simulink model "Joystick"  (Simulink 7.7)
settings: Solver=ode4  StartTime=0.0  StopTime=inf  FixedStep=sample_time  RelTol=1e-3
InitFcn:
  | sample_time=0.01;
libraries: vrlib x2, utility x1
settings Model: Creator=ttcl3  LastModifiedBy=CHIEW
settings SolverCC: MaxConsecutiveMinStep=auto
settings DebuggingCC: MultiTaskRateTransMsg=warning

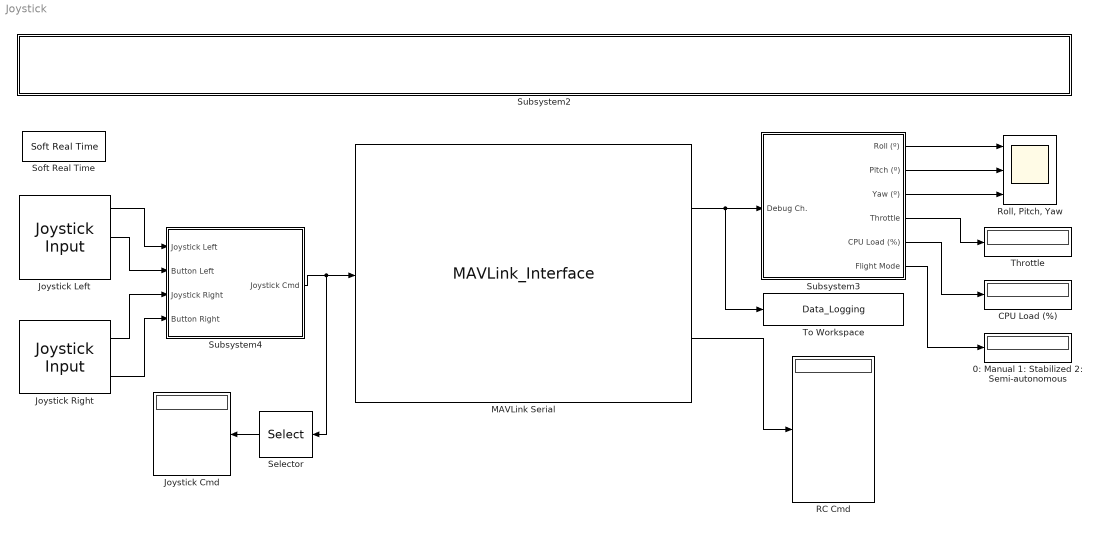
== system Joystick ==
  0: Manual 1: Stabilized 2: Semi-autonomous : Display
  CPU Load (%) : Display
  Joystick Cmd : Display
  Joystick Left : vrlib/Joystick Input  joyid=2  adjustports=on  forcefeed=off
  Joystick Right : vrlib/Joystick Input  joyid=1  adjustports=on  forcefeed=off
  MAVLink Serial : S-Function  FunctionName=MAVLink_Interface  Parameters=COM_Port,Baud_Rate,MSG_INPUT,MSG_OUTPUT  EnableBusSupport=off  mask{COM_Port='COM8', Baud_Rate=57600, HEART_BEAT=off, ATTITUDE_OUT=on, RAW_IMU=off, POSITION_OUT=off, VFR_HUD=off, RC_SCALED=on, SERVO_OUT_RAW=off, VICON_XYZ_RPY_Output=off, SET_MODE=off, DATA_STREAM=off, ATTITUDE_COMMAND=off, ATTITUDE_IN=off, GPS_RAW_IN=off, VFR_HUD_IN=off, VICON_XYZ_RPY=on, VICON_VEL=off, POSITION_DESIRED=off}
      mask prompts: COM_Port "COM Port"; Baud_Rate "Baud Rate"; HEART_BEAT "HEART BEAT"; ATTITUDE_OUT "ATTITUDE"; RAW_IMU "RAW IMU"; POSITION_OUT "GLOBAL POSITION"; VFR_HUD "VFR HUD"; RC_SCALED "RC CHANNELS SCALED"; SERVO_OUT_RAW "SERVO OUTPUT RAW"; VICON_XYZ_RPY_Output "VICON Output"; SET_MODE "SET MODE"; DATA_STREAM "REQUEST DATA STREAM"; ATTITUDE_COMMAND "ATTITUDE COMMAND"; ATTITUDE_IN "ATTITUDE (HIL)"; GPS_RAW_IN "GPS RAW (HIL)"; VFR_HUD_IN "AIRSPEED (HIL)"; VICON_XYZ_RPY "VICON POSITION"; VICON_VEL "VICON SPEED"; POSITION_DESIRED "Position Desired"
      mask init:
      | MSG_ID_NUM_INPUT = [uint8(11) uint8(66) uint8(59) uint8(30) uint8(32) uint8(73) uint8(104) uint8(103) uint8(50)];
      | MSG_ID_NAME_INPUT = [SET_MODE DATA_STREAM ATTITUDE_COMMAND ATTITUDE_IN GPS_RAW_IN VFR_HUD_IN VICON_XYZ_RPY VICON_VEL POSITION_DESIRED];
      | 
      | MSG_ID_NUM_OUTPUT = [uint8(0) uint8(30) uint8(27) uint8(73) uint8(74) uint8(34) uint8(37) uint8(104)];
      | MSG_ID_NAME_OUTPUT = [HEART_BEAT ATTITUDE_OUT RAW_IMU VFR_HUD POSITION_OUT RC_SCALED SERVO_OUT_RAW VICON_XYZ_RPY_Output];
      | 
      | idx_input = find(MSG_ID_NAME_INPUT);
      | MSG_INPUT = MSG_ID_NUM_INPUT(idx_input);
      | 
      | idx_output = find(MSG_ID_NAME_OUTPUT);
      | MSG_OUTPUT = MSG_ID_NUM_OUTPUT(idx_output);
      mask TabNameString: Setting,Setting,Output Message,Output Message,Output Message,Output Message,Output Message,Output Message,Output Message,Output Message,Input Message,Input Message,Input Message,Input Message,Input Message,Input Message,Input Message,Input Message,Input Message
      mask Display:
      | % Block image
      | image(imread('10-inch Quad Heat Map.png'));
      | 
      | %Label block
      | fprintf('MAVLink Serial\n%s\n%dbps', COM_Port,  Baud_Rate)
      | 
      | 
      | %Label input ports
      | 
      | in = 1;
      | if (SET_MODE == 1)
      |     port_label('input', in, 'SET MODE');
      |     in = in + 1;
      | end
      | if (DATA_STREAM == 1)
      |     port_label('input', in, 'REQUEST DATA STREAM');
      |     in = in + 1;
      | end
      | if (ATTITUDE_COMMAND == 1)
      |     port_label('input', in, 'ATTITUDE COMMAND');
      |     in = in + 1;
      | end
      | if (ATTITUDE_IN == 1)
      |     port_label('input', in, 'ATTITUDE (HIL)');
      |     in = in + 1;
      | end
      | if (GPS_RAW_IN == 1)
      |     port_label('input', in, 'GPS RAW (HIL)');
      |     in = in + 1;
      | end
      | if (VFR_HUD_IN == 1)
      |     port_label('input', in, 'AIRSPEED (HIL)');
      |     in = in + 1;
      | end
      | if (VICON_XYZ_RPY == 1)
      |     port_label('input', in, 'JOYSTICK CMD');
      |     in = in + 1;
      | end
      | if (VICON_VEL == 1)
      |     port_label('input', in, 'VICON_VEL');
      |     in = in + 1;
      | end
      | 
      | if (POSITION_DESIRED == 1)
      |     port_label('input', in, 'POSITION_DESIRED');
      |     in = in + 1;
      | end
      | 
      | %Label output ports
      | 
      | out = 1;
      | if (HEART_BEAT == 1)
      |     port_label('output', out, 'HEART BEAT');
      |     out = out + 1;
      | end
      | if (ATTITUDE_OUT == 1)
      |     port_label('output', out, 'DEBUG');
      |     out = out + 1;
      | end
      | if (RAW_IMU == 1)
      |     port_label('output', out, 'RAW IMU');
      |     out = out + 1;
      | end
      | if (POSITION_OUT == 1)
      |     port_label('output', out, 'GLOBAL POSITION');
      |     out = out + 1;
      | end
      | if (VFR_HUD == 1)
      |     port_label('output', out, 'VFR HUD');
      |     out = out + 1;
      | end
      | if (RC_SCALED == 1)
      |     port_label('output', out, 'RC CMD');
      |     out = out + 1;
      | end
      | if (SERVO_OUT_RAW == 1)
      |     port_label('output', out, 'SERVO OUTPUT RAW');
      |     out = out + 1;
      | end
      | % weihua, vicon output
      | if (VICON_XYZ_RPY_Output == 1)
      |     port_label('output', out, 'VICON_XYZ_RPY');
      |     out = out + 1;
      | end
  RC Cmd : Display
  "Roll, Pitch, Yaw" : Scope  NumInputPorts=3
      settings: TickLabels=on  TimeRange=24  YMin=-20~-10~-40  YMax=90~90~40  SampleInput=on
  Selector : Selector  InputPortWidth=7  IndexOptions=Index vector (dialog)  Indices=[4:7]  OutputSizes=1
  Soft Real Time : utility/Soft Real Time  x=0.8
  Subsystem2 : Subsystem
      mask Display:
      | %Label block
      | fprintf('NANYANG TECHNOLOGICAL UNIVERSITY')
  Subsystem3 : Subsystem
  Subsystem4 : Subsystem
  Throttle : Display
  To Workspace : ToWorkspace  VariableName=Data_Logging  SampleTime=-1  SaveFormat=Structure With Time
  wires:
  Subsystem4/1(Joystick Cmd) -> MAVLink Serial/1, Selector/1
  Joystick Left/1 -> Subsystem4/1(Joystick Left)
  Joystick Right/1 -> Subsystem4/3(Joystick Right)
  MAVLink Serial/2 -> RC Cmd/1
  Subsystem3/1(Roll (º)) -> "Roll, Pitch, Yaw"/1
  Subsystem3/2(Pitch (º)) -> "Roll, Pitch, Yaw"/2
  Subsystem3/3(Yaw (º)) -> "Roll, Pitch, Yaw"/3
  Subsystem3/4(Throttle) -> Throttle/1
  Subsystem3/5(CPU Load (%)) -> CPU Load (%)/1
  Subsystem3/6(Flight Mode) -> 0: Manual 1: Stabilized 2: Semi-autonomous/1
  Selector/1 -> Joystick Cmd/1
  MAVLink Serial/1 -> Subsystem3/1(Debug Ch.), To Workspace/1
  Joystick Right/2 -> Subsystem4/4(Button Right)
  Joystick Left/2 -> Subsystem4/2(Button Left)

== system Joystick/Subsystem2 ==

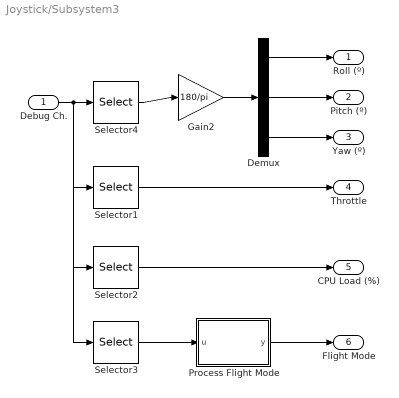
== system Joystick/Subsystem3 ==
  Debug Ch. : Inport
  Demux : Demux  Outputs=3
  Gain2 : Gain  Gain=180/pi
  Process Flight Mode : Stateflow chart  TreatAsAtomicUnit=on
  Selector1 : Selector  InputPortWidth=6  IndexOptions=Index vector (dialog)  Indices=4  OutputSizes=1
  Selector2 : Selector  InputPortWidth=6  IndexOptions=Index vector (dialog)  Indices=5  OutputSizes=1
  Selector3 : Selector  InputPortWidth=6  IndexOptions=Index vector (dialog)  Indices=6  OutputSizes=1
  Selector4 : Selector  InputPortWidth=6  IndexOptions=Index vector (dialog)  Indices=[1 2 3]  OutputSizes=1
  Roll (º) : Outport
  Pitch (º) : Outport  Port=2
  Yaw (º) : Outport  Port=3
  Throttle : Outport  Port=4
  CPU Load (%) : Outport  Port=5
  Flight Mode : Outport  Port=6
  wires:
  Selector4/1 -> Gain2/1
  Gain2/1 -> Demux/1
  Demux/1 -> Roll (º)/1
  Demux/2 -> Pitch (º)/1
  Debug Ch./1 -> Selector4/1, Selector1/1, Selector2/1, Selector3/1
  Demux/3 -> Yaw (º)/1
  Selector1/1 -> Throttle/1
  Selector2/1 -> CPU Load (%)/1
  Selector3/1 -> Process Flight Mode/1(u)
  Process Flight Mode/1(y) -> Flight Mode/1

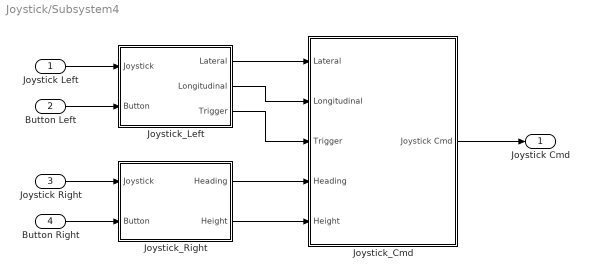
== system Joystick/Subsystem4 ==
  Joystick Left : Inport
  Button Left : Inport  Port=2
  Joystick Right : Inport  Port=3
  Button Right : Inport  Port=4
  Joystick_Cmd : Subsystem
  Joystick_Left : Subsystem
  Joystick_Right : Subsystem
  Joystick Cmd : Outport
  wires:
  Joystick_Right/2(Height) -> Joystick_Cmd/5(Height)
  Joystick_Left/1(Lateral) -> Joystick_Cmd/1(Lateral)
  Joystick Left/1 -> Joystick_Left/1(Joystick)
  Joystick_Cmd/1(Joystick Cmd) -> Joystick Cmd/1
  Joystick Right/1 -> Joystick_Right/1(Joystick)
  Button Right/1 -> Joystick_Right/2(Button)
  Joystick_Left/2(Longitudinal) -> Joystick_Cmd/2(Longitudinal)
  Joystick_Right/1(Heading) -> Joystick_Cmd/4(Heading)
  Button Left/1 -> Joystick_Left/2(Button)
  Joystick_Left/3(Trigger) -> Joystick_Cmd/3(Trigger)

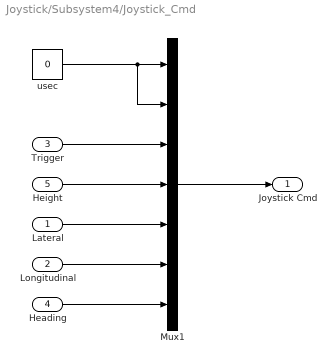
== system Joystick/Subsystem4/Joystick_Cmd ==
  Lateral : Inport
  Longitudinal : Inport  Port=2
  Trigger : Inport  Port=3
  Heading : Inport  Port=4
  Height : Inport  Port=5
  Mux1 : Mux  Inputs=7
  usec : Constant  Value=0  SampleTime=sample_time
  Joystick Cmd : Outport
  wires:
  usec/1 -> Mux1/1, Mux1/2
  Mux1/1 -> Joystick Cmd/1
  Height/1 -> Mux1/4
  Lateral/1 -> Mux1/5
  Longitudinal/1 -> Mux1/6
  Heading/1 -> Mux1/7
  Trigger/1 -> Mux1/3

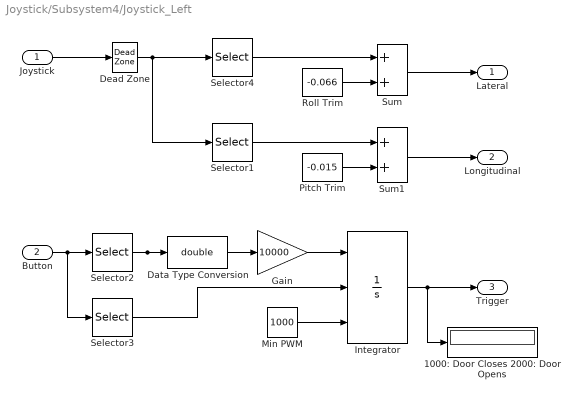
== system Joystick/Subsystem4/Joystick_Left ==
  Joystick : Inport
  Button : Inport  Port=2
  1000: Door Closes 2000: Door Opens : Display
  Data Type Conversion : DataTypeConversion  OutDataTypeStr=double
  Dead Zone : DeadZone  LowerValue=-0.1  UpperValue=0.1  SaturateOnIntegerOverflow=on
  Gain : Gain  Gain=10000
  Integrator : Integrator  ExternalReset=either  InitialConditionSource=external  LimitOutput=on  UpperSaturationLimit=1800  LowerSaturationLimit=1000
  Min PWM : Constant  Value=1000
  Pitch Trim : Constant  Value=-0.015
  Roll Trim : Constant  Value=-0.066
  Selector1 : Selector  InputPortWidth=4  IndexOptions=Index vector (dialog)  Indices=2  OutputSizes=1
  Selector2 : Selector  InputPortWidth=12  IndexOptions=Index vector (dialog)  Indices=1  OutputSizes=1
  Selector3 : Selector  InputPortWidth=12  IndexOptions=Index vector (dialog)  Indices=4  OutputSizes=1
  Selector4 : Selector  InputPortWidth=4  IndexOptions=Index vector (dialog)  Indices=1  OutputSizes=1
  Sum : Sum
  Sum1 : Sum
  Lateral : Outport
  Longitudinal : Outport  Port=2
  Trigger : Outport  Port=3
  wires:
  Joystick/1 -> Dead Zone/1
  Roll Trim/1 -> Sum/2
  Pitch Trim/1 -> Sum1/2
  Dead Zone/1 -> Selector4/1, Selector1/1
  Selector4/1 -> Sum/1
  Selector1/1 -> Sum1/1
  Sum/1 -> Lateral/1
  Sum1/1 -> Longitudinal/1
  Button/1 -> Selector2/1, Selector3/1
  Selector2/1 -> Data Type Conversion/1
  Min PWM/1 -> Integrator/3
  Data Type Conversion/1 -> Gain/1
  Gain/1 -> Integrator/1
  Selector3/1 -> Integrator/2
  Integrator/1 -> Trigger/1, 1000: Door Closes 2000: Door Opens/1

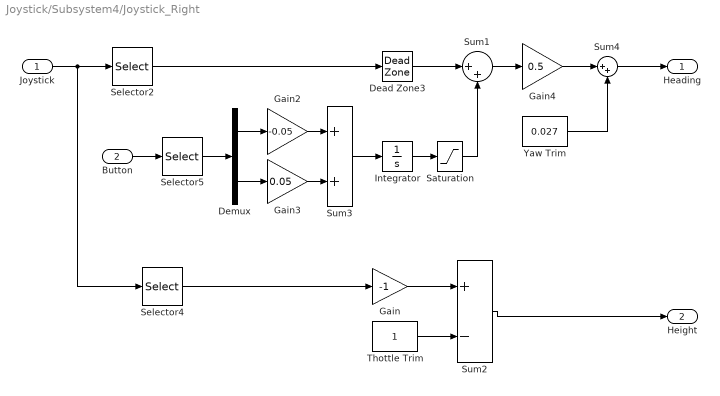
== system Joystick/Subsystem4/Joystick_Right ==
  Joystick : Inport
  Button : Inport  Port=2
  Dead Zone3 : DeadZone  LowerValue=-0.2  UpperValue=0.2  SaturateOnIntegerOverflow=on
  Demux : Demux  Outputs=2
  Gain : Gain  Gain=-1
  Gain2 : Gain  Gain=-0.05
  Gain3 : Gain  Gain=0.05
  Gain4 : Gain  Gain=0.5
  Integrator : Integrator
  Saturation : Saturate  UpperLimit=0.1  LowerLimit=-0.1
  Selector2 : Selector  InputPortWidth=3  IndexOptions=Index vector (dialog)  Indices=[1]  OutputSizes=1
  Selector4 : Selector  InputPortWidth=3  IndexOptions=Index vector (dialog)  Indices=2  OutputSizes=1
  Selector5 : Selector  InputPortWidth=11  IndexOptions=Index vector (dialog)  Indices=[4 5]  OutputSizes=1
  Sum1 : Sum  Inputs=|++
  Sum2 : Sum  Inputs=+-
  Sum3 : Sum  OutDataTypeStr=double
  Sum4 : Sum  Inputs=|++
  Thottle Trim : Constant
  Yaw Trim : Constant  Value=0.027
  Heading : Outport
  Height : Outport  Port=2
  wires:
  Selector2/1 -> Dead Zone3/1
  Selector4/1 -> Gain/1
  Joystick/1 -> Selector2/1, Selector4/1
  Gain/1 -> Sum2/1
  Thottle Trim/1 -> Sum2/2
  Sum2/1 -> Height/1
  Button/1 -> Selector5/1
  Selector5/1 -> Demux/1
  Demux/2 -> Gain3/1
  Demux/1 -> Gain2/1
  Gain2/1 -> Sum3/1
  Gain3/1 -> Sum3/2
  Sum3/1 -> Integrator/1
  Dead Zone3/1 -> Sum1/1
  Integrator/1 -> Saturation/1
  Saturation/1 -> Sum1/2
  Gain4/1 -> Sum4/1
  Yaw Trim/1 -> Sum4/2
  Sum4/1 -> Heading/1
  Sum1/1 -> Gain4/1

== matlab function Subsystem3/Process Flight Mode ==
  data: u input double; y output double
function y = fcn(u)
%#codegen

if u <=-0.5
    y = 0;  % Manual
elseif u>=0.5
    y = 2;  % Semi-autonomous
else
    y = 1;  % Stabilized
end
